simulink model "pomper_m"  (Simulink 7.9)
settings: Solver=ode45  SolverMode=SingleTasking  StartTime=0.0  StopTime=999999  MaxStep=10  RelTol=1e-3  AbsTol=1e-3
values from neighbouring files (symbols this model uses):
  U = st_Varia('LongNames')    [pomper_i.m]
  x0 = []    [pomper_i.m]    (also in pomper_s.m = x0)
undefined symbols (not defined in the file or in its folder): B
settings Model: Creator=M.Sparnaaij  LastModifiedBy=M.Sparnaaij
settings DataIOCC: LimitDataPoints=off  SaveOutput=off  SaveTime=off  SignalLoggingName=sigsOut
settings OptimizationCC: BooleanDataType=off
settings DebuggingCC: SaveWithParameterizedLinksMsg=none  SignalResolutionControl=TryResolveAllWithWarning  SolverPrmCheckMsg=none  MultiTaskDSMMsg=warning  MultiTaskCondExecSysMsg=none  StrictBusMsg=None
settings HardwareCC: TargetUnknown=on
settings RTWCC: IncludeERTFirstTime=on
settings GRTTargetCC: CombineOutputUpdateFcns=off  GRTInterface=on

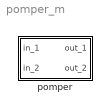
== system pomper_m ==
  pomper : Subsystem  Description=pomper
      mask init:
      | filenaam='.\StimelaData\pomper_p.mat';
      | 
      | [Pn,Fn,Fext]=Fileprop(filenaam);
      | 
      | errstr = st_UniqName(filenaam,'filenaam=''','SubSystem','OpenFcn');
      | if errstr, error([errstr 'The filename "' filenaam '" is already in use. Choose a different filename.']), end
      | 
      | P = pomper_p(filenaam);
      | [B,x0,U]=pomper_i(filenaam);
      settings: OpenFcn=|
      | filenaam='.\StimelaData\pomper_p.mat';
      | st_ParameterInput('init',gcb,filenaam,'pomper');
      mask Display:
      | plot(0,0,100,100,[0 20],[80 80],[0 20],[85 85],[0 20],[20 20],[80 100],[80 80],[80 100],[85 85],[80 100],[ 20 20],[80 100],[ 15 15],[20 80 80 20 20],[10 10 90  90 10]);
      | disp('')
      | text(50,50,'pomper', 'horizontalAlignment', 'center', 'verticalAlignment', 'middle');
      | text(50,0,Fn, 'horizontalAlignment', 'center', 'verticalAlignment', 'base');

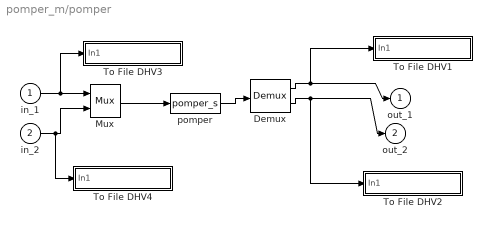
== system pomper_m/pomper ==
  in_1 : Inport
  in_2 : Inport  Port=2
  Demux : Demux  Outputs=[U.Number B.Measurements]
  Mux : Mux  Inputs=[U.Number B.Setpoints]
  To File DHV1 : Subsystem  mask(To File DHV){naam=[filenaam(1:length(filenaam)-4) '_out.sti']}
      mask prompts: naam "Naam van bestand"
      mask init:
      | set_param([gcb '/To File'],'Filename',naam);
      mask Display: disp(naam)
  To File DHV2 : Subsystem  mask(To File DHV){naam=[filenaam(1:length(filenaam)-4) '_EM.sti']}
      mask prompts: naam "Naam van bestand"
      mask init:
      | set_param([gcb '/To File'],'Filename',naam);
      mask Display: disp(naam)
  To File DHV3 : Subsystem  mask(To File DHV){naam=[filenaam(1:length(filenaam)-4) '_in.sti']}
      mask prompts: naam "Naam van bestand"
      mask init:
      | set_param([gcb '/To File'],'Filename',naam);
      mask Display: disp(naam)
  To File DHV4 : Subsystem  mask(To File DHV){naam=[filenaam(1:length(filenaam)-4) '_ES.sti']}
      mask prompts: naam "Naam van bestand"
      mask init:
      | set_param([gcb '/To File'],'Filename',naam);
      mask Display: disp(naam)
  pomper : S-Function  FunctionName=pomper_s  Parameters=B,x0,U,P  EnableBusSupport=off
  out_1 : Outport  InitialOutput=0
  out_2 : Outport  Port=2  InitialOutput=0
  wires:
  in_2/1 -> To File DHV4/1(In1), Mux/2
  Mux/1 -> pomper/1
  in_1/1 -> To File DHV3/1(In1), Mux/1
  pomper/1 -> Demux/1
  Demux/1 -> To File DHV1/1(In1), out_1/1
  Demux/2 -> To File DHV2/1(In1), out_2/1

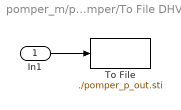
== system pomper_m/pomper/To File DHV1 ==
  In1 : Inport
  To File : ToFile  Filename=./pomper_p_out.sti  MatrixName=pomperout
  wires:
  In1/1 -> To File/1

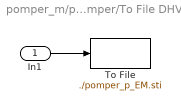
== system pomper_m/pomper/To File DHV2 ==
  In1 : Inport
  To File : ToFile  Filename=./pomper_p_EM.sti  MatrixName=pomperEM
  wires:
  In1/1 -> To File/1

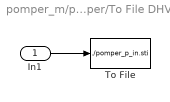
== system pomper_m/pomper/To File DHV3 ==
  In1 : Inport
  To File : ToFile  Filename=./pomper_p_in.sti  MatrixName=pomperin
  wires:
  In1/1 -> To File/1

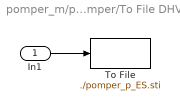
== system pomper_m/pomper/To File DHV4 ==
  In1 : Inport
  To File : ToFile  Filename=./pomper_p_ES.sti  MatrixName=pomperES
  wires:
  In1/1 -> To File/1
